simulink model "TMATS_Example_2"  (R2019a)
settings: Solver=VariableStepAuto  StartTime=0.0  StopTime=10.0  RelTol=1e-3
undefined symbols (not defined in the file): stripchar_TMATS
libraries: Lib_Turbo_Ambient_TMATS x1, Lib_Turbo_Burner_TMATS x1, Lib_Turbo_Compressor_TMATS x1, Lib_Turbo_Duct_TMATS x1, Lib_Turbo_Nozzle_TMATS x1, Lib_Turbo_Shaft_TMATS x1, Lib_Turbo_Turbine_TMATS x1
settings Model: Creator=bbraunj  LastModifiedBy=bbraunj

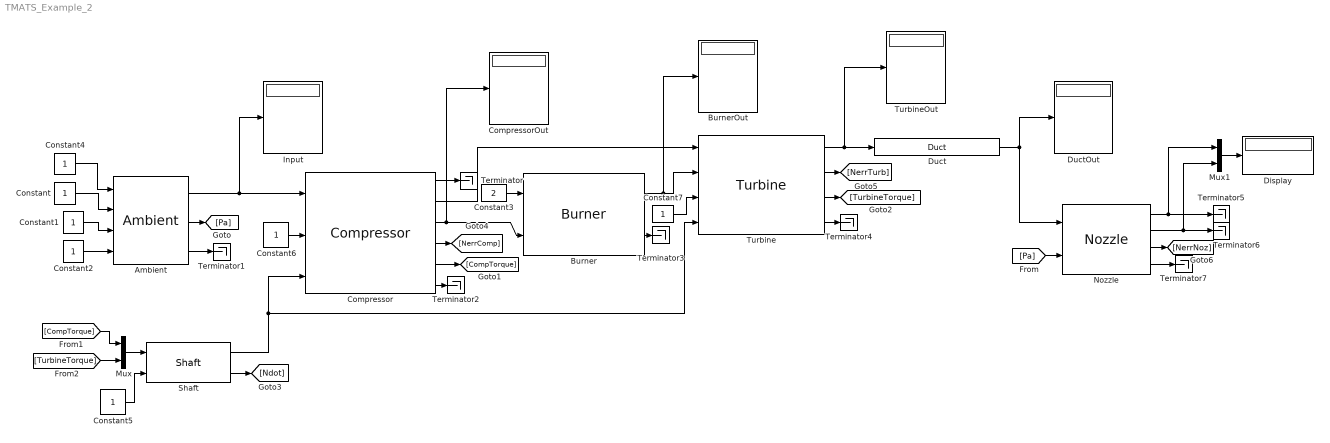
== system TMATS_Example_2 ==
  Ambient : Lib_Turbo_Ambient_TMATS/Ambient  X_A_AltVec_M=5000*[-1 0 1 2 3 4 5 6 7 8 9 10 12 14 16]  T_A_TsVec_M=[536.51 518.67 500.84 483.03 465.22 447.41 429.62 411.84 394.06 389.97 389.97 389.97 389.97 392.25 397.69]  T_A_PsVec_M=[17.554 14.696 12.228 10.108 8.297 6.759 5.461 4.373 3.468 2.73 2.149 1.692 1.049 0.651 0.406]  AFARc_M=0  X_A_FARVec_M=[0; 0.0050; 0.0100; 0.0150; 0.0200; 0.0250; 0.0300]  T_A_RtArray_M="[0.0686;    0.0686;    0.0686;    0.0686;    0.0686;    0.0686;    0.0686]"  Y_A_TVec_M=[300 10000]  T_A_gammaArray_M=[ 1.4 1.4 1.4 1.4 1.4 1.4 1.4; 1.4 1.4 1.4 1.4 1.4 1.4 1.4]
  Burner : Lib_Turbo_Burner_TMATS/Burner  LHVEn_M=on  LHV_M=18400  Eff_M=1  hFuel_M=-1200  dPnormBurner_M=0.05
  BurnerOut : Display
  Compressor : Lib_Turbo_Compressor_TMATS/Compressor  X_C_RlineVec_M=[1.000 3.000 ]  Z_C_AlphaVec_M=1  Y_C_Map_NcVec_M="[0.500  0.900  1.050]"  T_C_Map_WcArray_M=[0 0; 0 0; 0 0]  T_C_Map_PRArray_M=[0 0; 0 0; 0 0]  T_C_Map_EffArray_M=[0 0; 0 0; 0 0]  s_C_Nc_M=0.0001  s_C_Wc_M=0.4953  s_C_PR_M=0.8636  s_C_Eff_M=0.9977  SL_M=off  Scale_M=none  CBLDEN_M=off  C_CBD_M=0  C_CBFht_M=0.5  C_CBFPt_M=0.5  FBLDEN_M=off  C_FBD_M=0  C_BFht_M=0.5  C_BFPt_M=0.5  DefSMEn_M=on  SRline_M=1  X_C_Map_WcSurgeVec_M=[0 200]  T_C_Map_PRSurgeVec_M=[30 30]  iDesign_M=2  NcDes_M=10000  EffDes_M=0.95  PRDes_M=20  RlineDes_M=2  FVar_M=strcat('iDes_',stripchar_TMATS(gcb),'.bin')  BlkNm_M=double(gcb)  HP_M=off
  CompressorOut : Display
  Constant{,1..2,4..7} (7 alike) : Constant
  Constant3 : Constant  Value=2
  Display : Display
  Duct : Lib_Turbo_Duct_TMATS/Duct  dP_M=0.005
  DuctOut : Display
  Input : Display
  Mux : Mux  Inputs=2
  Mux1 : Mux  Inputs=2
  Nozzle : Lib_Turbo_Nozzle_TMATS/Nozzle  SWType_M=Convergent  N_TArea_M=110.7  N_EArea_M=110.7  N_FL_M=0.00  X_N_TtVec2_M=[300 10000]  T_N_TGArray_M=[1 1]  X_N_PEQPaVec_M=[0 10000]  T_N_CdThArray_M=[1 1]  T_N_CvArray_M=[0.990 0.990]  CfgEn_M=off  T_N_CfgArray_M=[1 1]  X_N_FARVec_M=[0; 0.0050; 0.0100; 0.0150; 0.0200; 0.0250; 0.0300]  T_N_RtArray_M="[0.0686;    0.0686;    0.0686;    0.0686;    0.0686;    0.0686;    0.0686]"  Y_N_TtVec_M=[300 10000]  T_N_MAP_gammaArray_M=[ 1.4 1.4 1.4 1.4 1.4 1.4 1.4; 1.4 1.4 1.4 1.4 1.4 1.4 1.4]  iDesign_M=2  WDes_M=100  FVar_M=strcat('iDes_',stripchar_TMATS(gcb),'.bin')
  Shaft : Lib_Turbo_Shaft_TMATS/Shaft  Shaft_Inertia_M=0.3183
  Terminator{,1..7} (8 alike) : Terminator
  Turbine : Lib_Turbo_Turbine_TMATS/Turbine  X_T_Map_PRVec_M="[ 3.000  8.000]"  Y_T_Map_NcVec_M="[60 80  110]"  T_T_Map_WcArray_M=[0 0;0 0; 0 0]  T_T_Map_EffArray_M=[0 0; 0 0; 0 0]  s_T_Nc_M=0.0243  s_T_Wc_M=0.4504  s_T_PR_M=0.9736  s_T_Eff_M=0.9984  ConfigNPSS_M=0  Scale_M=none  CFlwEn_M=off  T_CoolFlwPos_M=0  iDesign_M=2  NcDes_M=100  EffDes_M=0.9328  PRDes_M=5  NDes_M=10000  FVar_M=strcat('iDes_',stripchar_TMATS(gcb),'.bin')  BlkNm_M=double(gcb)  HP_M=off
  TurbineOut : Display
  wires:
  Duct/1 -> Nozzle/1, DuctOut/1
  Compressor/3 -> Burner/2, CompressorOut/1
  Burner/1 -> BurnerOut/1, Turbine/2
  Turbine/1 -> TurbineOut/1, Duct/1
  Compressor/2 -> Turbine/1
  Compressor/1 -> Terminator/1
  Shaft/1 -> Compressor/3, Turbine/4
  Mux/1 -> Shaft/1
  Ambient/1 -> Input/1, Compressor/1
  Ambient/3 -> Terminator1/1
  Constant/1 -> Ambient/2
  Constant1/1 -> Ambient/3
  Constant2/1 -> Ambient/4
  Ambient/2 -> [Pa]
  [Pa] -> Nozzle/2
  Compressor/5 -> [CompTorque]
  [CompTorque] -> Mux/1
  [TurbineTorque] -> Mux/2
  Turbine/3 -> [TurbineTorque]
  Constant3/1 -> Burner/1
  Compressor/6 -> Terminator2/1
  Burner/2 -> Terminator3/1
  Turbine/4 -> Terminator4/1
  Nozzle/2 -> Mux1/2, Terminator6/1
  Nozzle/1 -> Mux1/1, Terminator5/1
  Nozzle/4 -> Terminator7/1
  Mux1/1 -> Display/1
  Constant4/1 -> Ambient/1
  Constant5/1 -> Shaft/2
  Shaft/2 -> [Ndot]
  Constant6/1 -> Compressor/2
  Compressor/4 -> [NerrComp]
  Constant7/1 -> Turbine/3
  Turbine/2 -> [NerrTurb]
  Nozzle/3 -> [NerrNoz]
